simulink model "SIFT"  (R2013a)
settings: Solver=FixedStepDiscrete  SolverMode=SingleTasking  StartTime=0.0  StopTime=10.0  RelTol=1e-3
libraries: xbsIndex_r4 x365, xrbsImage_r4 x64
(part 1 of 10)
settings Model: Creator=Gururaja  LastModifiedBy=Gururaja
settings DataIOCC: SignalLogging=off
settings OptimizationCC: BlockReduction=off  ConditionallyExecuteInputs=off  InlineParams=on
settings DebuggingCC: AlgebraicLoopMsg=error
settings HardwareCC: ProdHWDeviceType=ASIC/FPGA->ASIC/FPGA  ProdEqTarget=off

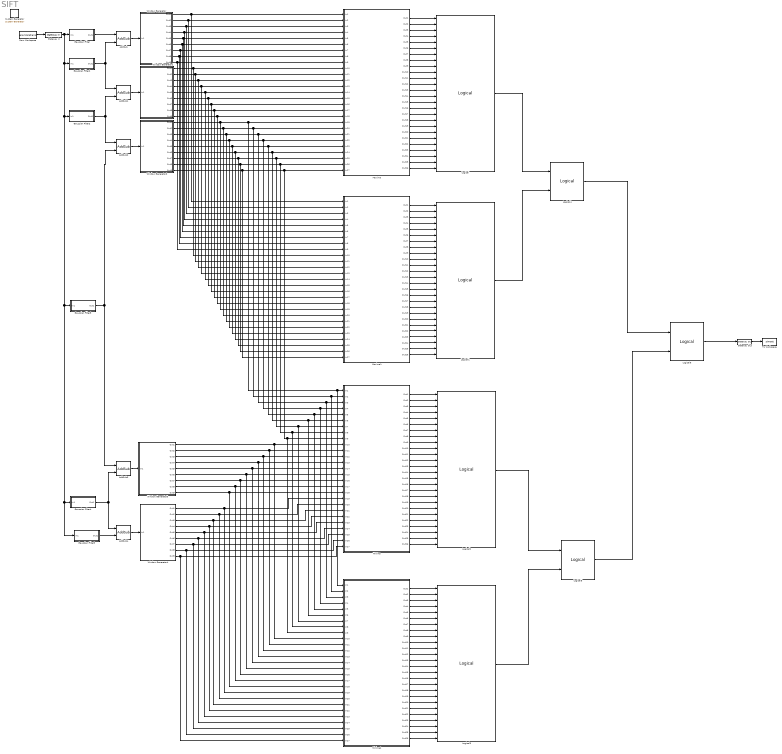
== system SIFT ==
  " System Generator" : xbsIndex_r4/ System Generator  Tag=genX  xilinxfamily=virtex5  part=xc5vsx50t  speed=-1  package=ff1136  synthesis_tool=XST  clock_wrapper=Clock Enables  directory=./netlist  proj_type=Project Navigator  Synth_file=XST Defaults  Impl_file=ISE Defaults  testbench=off  simulink_period=1  sysclk_period=10  dcm_input_clock_period=10  incr_netlist=off  trim_vbits=Everywhere in SubSystem  dbl_ovrd=According to Block Masks  core_generation=According to Block Masks  run_coregen=off  deprecated_control=off  eval_field=0  block_type=sysgen
  AddSub{,1..4} (5 alike) : xbsIndex_r4/AddSub  mode=Subtraction  use_carryin=off  use_carryout=off  en=off  latency=0  precision=User Defined  arith_type=Unsigned  n_bits=8  bin_pt=0  quantization="Round  (unbiased: +/- Inf)"  overflow=Saturate  dbl_ovrd=off  use_behavioral_HDL=off  hw_selection=Fabric  pipelined=off  block_type=addsub
  From Workspace : FromWorkspace  VariableName=grayScaleSignal  SampleTime=1  Interpolate=off  OutputAfterFinalValue=Setting to zero
  Gateway In : xbsIndex_r4/Gateway In  gui_display_data_type=Fixed-point  arith_type=Unsigned  n_bits=8  bin_pt=0  preci_type=Single  exp_width=8  frac_width=24  quantization="Round  (unbiased: +/- Inf)"  overflow=Saturate  period=1  dbl_ovrd=off  timing_constraint=None  locs_specified=off  LOCs={}  UseAsADC=off  ADCChannel='1'  inherit_from_input=off  hdl_port=on  block_type=gatewayin
  Gateway Out : xbsIndex_r4/Gateway Out  inherit_from_input=off  hdl_port=on  timing_constraint="Data Rate;  Set 'FAST' Attribute"  locs_specified=off  LOCs={}  UseAsDAC=off  DACChannel='1'  block_type=gatewayout
  Gaussian Filter : Subsystem
  Gaussian Filter1 : Subsystem
  Gaussian Filter2 : Subsystem
  Gaussian Filter3 : Subsystem
  Gaussian Filter4 : Subsystem
  Gaussian Filter5 : Subsystem
  Logical{,1..3} (4 alike) : xbsIndex_r4/Logical  logical_function=AND  inputs=26  en=off  latency=1  precision=User Defined  arith_type=Unsigned  n_bits=8  bin_pt=0  align_bp=on  dbl_ovrd=off  block_type=logical
  Logical4 : xbsIndex_r4/Logical  logical_function=OR  inputs=2  en=off  latency=1  precision=Full  arith_type=Unsigned  n_bits=16  bin_pt=0  align_bp=on  dbl_ovrd=off  block_type=logical
  Logical5 : xbsIndex_r4/Logical  logical_function=OR  inputs=2  en=off  latency=1  precision=Full  arith_type=Unsigned  n_bits=16  bin_pt=0  align_bp=on  dbl_ovrd=off  block_type=logical
  Logical6 : xbsIndex_r4/Logical  logical_function=OR  inputs=2  en=off  latency=1  precision=Full  arith_type=Unsigned  n_bits=16  bin_pt=0  align_bp=on  dbl_ovrd=off  block_type=logical
  Maxima : Subsystem
  Maxima1 : Subsystem
  Minima : Subsystem
  Minima1 : Subsystem
  To Workspace : ToWorkspace  VariableName=simout  SampleTime=1
  Window Generator : Subsystem
  Window Generator1 : Subsystem
  Window Generator2 : Subsystem
  Window Generator3 : Subsystem
  Window Generator4 : Subsystem
  wires:
  From Workspace/1 -> Gateway In/1
  Gateway In/1 -> Gaussian Filter1/1(In1), Gaussian Filter2/1(In1), Gaussian Filter3/1(In1), Gaussian Filter5/1(In1), Gaussian Filter4/1(In1), Gaussian Filter/1(In1)
  AddSub/1 -> Window Generator/1(In1)
  AddSub1/1 -> Window Generator1/1(In1)
  AddSub2/1 -> Window Generator2/1(In1)
  AddSub3/1 -> Window Generator3/1(In1)
  AddSub4/1 -> Window Generator4/1(In1)
  Window Generator/1(Out1) -> Maxima1/1(In1), Maxima/1(In1)
  Window Generator/3(Out3) -> Maxima1/3(In3), Maxima/3(In3)
  Window Generator/4(Out4) -> Maxima1/4(In4), Maxima/4(In4)
  Window Generator/5(Out5) -> Maxima1/5(In5), Maxima/5(In5)
  Window Generator/6(Out6) -> Maxima1/6(In6), Maxima/6(In6)
  Window Generator/7(Out7) -> Maxima1/7(In7), Maxima/7(In7)
  Window Generator/8(Out8) -> Maxima1/8(In8), Maxima/8(In8)
  Window Generator/9(Out9) -> Maxima1/9(In9), Maxima/9(In9)
  Window Generator1/1(Out1) -> Maxima1/10(In10), Maxima/10(In10)
  Window Generator1/2(Out2) -> Maxima1/11(In11), Maxima/11(In11)
  Window Generator1/3(Out3) -> Maxima1/12(In12), Maxima/12(In12)
  Window Generator1/4(Out4) -> Maxima1/13(In13), Maxima/13(In13)
  Window Generator1/5(Out5) -> Maxima1/14(In14), Maxima/14(In14)
  Window Generator1/6(Out6) -> Maxima1/15(In15), Maxima/15(In15)
  Window Generator1/7(Out7) -> Maxima1/16(In16), Maxima/16(In16)
  Window Generator1/8(Out8) -> Maxima1/17(In17), Maxima/17(In17)
  Window Generator1/9(Out9) -> Maxima1/18(In18), Maxima/18(In18)
  Window Generator2/1(Out1) -> Maxima1/19(In19), Minima1/1(In1), Minima/1(In1), Maxima/19(In19)
  Window Generator2/2(Out2) -> Maxima1/20(In20), Minima1/2(In2), Minima/2(In2), Maxima/20(In20)
  Window Generator2/3(Out3) -> Maxima1/21(In21), Minima1/3(In3), Minima/3(In3), Maxima/21(In21)
  Window Generator2/4(Out4) -> Maxima1/22(In22), Minima1/4(In4), Minima/4(In4), Maxima/22(In22)
  Window Generator2/5(Out5) -> Maxima1/23(In23), Minima1/5(In5), Minima/5(In5), Maxima/23(In23)
  Window Generator2/6(Out6) -> Maxima1/24(In24), Minima1/6(In6), Minima/6(In6), Maxima/24(In24)
  Window Generator2/7(Out7) -> Maxima1/25(In25), Minima1/7(In7), Minima/7(In7), Maxima/25(In25)
  Window Generator2/8(Out8) -> Maxima1/26(In26), Minima1/8(In8), Minima/8(In8), Maxima/26(In26)
  Window Generator2/9(Out9) -> Maxima1/27(In27), Minima1/9(In9), Minima/9(In9), Maxima/27(In27)
  Window Generator/2(Out2) -> Maxima1/2(In2), Maxima/2(In2)
  Window Generator3/1(Out1) -> Minima1/10(In10), Minima/10(In10)
  Window Generator3/2(Out2) -> Minima1/11(In11), Minima/11(In11)
  Window Generator3/3(Out3) -> Minima1/12(In12), Minima/12(In12)
  Window Generator3/4(Out4) -> Minima1/13(In13), Minima/13(In13)
  Window Generator3/5(Out5) -> Minima1/14(In14), Minima/14(In14)
  Window Generator3/6(Out6) -> Minima1/15(In15), Minima/15(In15)
  Window Generator3/7(Out7) -> Minima1/16(In16), Minima/16(In16)
  Window Generator3/8(Out8) -> Minima1/17(In17), Minima/17(In17)
  Window Generator3/9(Out9) -> Minima1/18(In18), Minima/18(In18)
  Window Generator4/1(Out1) -> Minima1/19(In19), Minima/19(In19)
  Window Generator4/2(Out2) -> Minima1/20(In20), Minima/20(In20)
  Window Generator4/3(Out3) -> Minima1/21(In21), Minima/21(In21)
  Window Generator4/4(Out4) -> Minima1/22(In22), Minima/22(In22)
  Window Generator4/5(Out5) -> Minima1/23(In23), Minima/23(In23)
  Window Generator4/6(Out6) -> Minima1/24(In24), Minima/24(In24)
  Window Generator4/7(Out7) -> Minima1/25(In25), Minima/25(In25)
  Window Generator4/8(Out8) -> Minima1/26(In26), Minima/26(In26)
  Window Generator4/9(Out9) -> Minima1/27(In27), Minima/27(In27)
  Maxima/1(Out1) -> Logical/1
  Maxima/2(Out2) -> Logical/2
  Maxima/3(Out3) -> Logical/3
  Maxima/4(Out4) -> Logical/4
  Maxima/5(Out5) -> Logical/5
  Maxima/6(Out6) -> Logical/6
  Maxima/7(Out7) -> Logical/7
  Maxima/8(Out8) -> Logical/8
  Maxima/9(Out9) -> Logical/9
  Maxima/10(Out10) -> Logical/10
  Maxima/11(Out11) -> Logical/11
  Maxima/12(Out12) -> Logical/12
  Maxima/13(Out13) -> Logical/13
  Maxima/14(Out14) -> Logical/14
  Maxima/15(Out15) -> Logical/15
  Maxima/16(Out16) -> Logical/16
  Maxima/17(Out17) -> Logical/17
  Maxima/18(Out18) -> Logical/18
  Maxima/19(Out19) -> Logical/19
  Maxima/20(Out20) -> Logical/20
  Maxima/21(Out21) -> Logical/21
  Maxima/22(Out22) -> Logical/22
  Maxima/23(Out23) -> Logical/23
  Maxima/24(Out24) -> Logical/24
  Maxima/25(Out25) -> Logical/25
  Maxima/26(Out26) -> Logical/26
  Maxima1/1(Out1) -> Logical1/1
  Maxima1/2(Out2) -> Logical1/2
  Maxima1/3(Out3) -> Logical1/3
  Maxima1/4(Out4) -> Logical1/4
  Maxima1/5(Out5) -> Logical1/5
  Maxima1/6(Out6) -> Logical1/6
  Maxima1/7(Out7) -> Logical1/7
  Maxima1/8(Out8) -> Logical1/8
  Maxima1/9(Out9) -> Logical1/9
  Maxima1/10(Out10) -> Logical1/10
  Maxima1/11(Out11) -> Logical1/11
  Maxima1/12(Out12) -> Logical1/12
  Maxima1/13(Out13) -> Logical1/13
  Maxima1/14(Out14) -> Logical1/14
  Maxima1/15(Out15) -> Logical1/15
  Maxima1/16(Out16) -> Logical1/16
  Maxima1/17(Out17) -> Logical1/17
  Maxima1/18(Out18) -> Logical1/18
  Maxima1/19(Out19) -> Logical1/19
  Maxima1/20(Out20) -> Logical1/20
  Maxima1/21(Out21) -> Logical1/21
  Maxima1/22(Out22) -> Logical1/22
  Maxima1/23(Out23) -> Logical1/23
  Maxima1/24(Out24) -> Logical1/24
  Maxima1/25(Out25) -> Logical1/25
  Maxima1/26(Out26) -> Logical1/26
  Minima/1(Out1) -> Logical2/1
  Minima/2(Out2) -> Logical2/2
  Minima/3(Out3) -> Logical2/3
  Minima/4(Out4) -> Logical2/4
  Minima/5(Out5) -> Logical2/5
  Minima/6(Out6) -> Logical2/6
  Minima/7(Out7) -> Logical2/7
  Minima/8(Out8) -> Logical2/8
  Minima/9(Out9) -> Logical2/9
  Minima/10(Out10) -> Logical2/10
  Minima/11(Out11) -> Logical2/11
  Minima/12(Out12) -> Logical2/12
  Minima/13(Out13) -> Logical2/13
  Minima/14(Out14) -> Logical2/14
  Minima/15(Out15) -> Logical2/15
  Minima/16(Out16) -> Logical2/16
  Minima/17(Out17) -> Logical2/17
  Minima/18(Out18) -> Logical2/18
  Minima/19(Out19) -> Logical2/19
  Minima/20(Out20) -> Logical2/20
  Minima/21(Out21) -> Logical2/21
  Minima/22(Out22) -> Logical2/22
  Minima/23(Out23) -> Logical2/23
  Minima/24(Out24) -> Logical2/24
  Minima/25(Out25) -> Logical2/25
  Minima/26(Out26) -> Logical2/26
  Minima1/1(Out1) -> Logical3/1
  Minima1/2(Out2) -> Logical3/2
  Minima1/3(Out3) -> Logical3/3
  Minima1/4(Out4) -> Logical3/4
  Minima1/5(Out5) -> Logical3/5
  Minima1/6(Out6) -> Logical3/6
  Minima1/7(Out7) -> Logical3/7
  Minima1/8(Out8) -> Logical3/8
  Minima1/9(Out9) -> Logical3/9
  Minima1/10(Out10) -> Logical3/10
  Minima1/11(Out11) -> Logical3/11
  Minima1/12(Out12) -> Logical3/12
  Minima1/13(Out13) -> Logical3/13
  Minima1/14(Out14) -> Logical3/14
  Minima1/15(Out15) -> Logical3/15
  Minima1/16(Out16) -> Logical3/16
  Minima1/17(Out17) -> Logical3/17
  Minima1/18(Out18) -> Logical3/18
  Minima1/19(Out19) -> Logical3/19
  Minima1/20(Out20) -> Logical3/20
  Minima1/21(Out21) -> Logical3/21
  Minima1/22(Out22) -> Logical3/22
  Minima1/23(Out23) -> Logical3/23
  Minima1/24(Out24) -> Logical3/24
  Minima1/25(Out25) -> Logical3/25
  Minima1/26(Out26) -> Logical3/26
  Logical/1 -> Logical4/1
  Logical1/1 -> Logical4/2
  Logical2/1 -> Logical5/1
  Logical3/1 -> Logical5/2
  Logical4/1 -> Logical6/1
  Logical5/1 -> Logical6/2
  Logical6/1 -> Gateway Out/1
  Gateway Out/1 -> To Workspace/1
  Gaussian Filter/1(Out1) -> AddSub/1
  Gaussian Filter1/1(Out1) -> AddSub/2, AddSub1/1
  Gaussian Filter2/1(Out1) -> AddSub2/1, AddSub1/2
  Gaussian Filter3/1(Out1) -> AddSub2/2, AddSub3/1
  Gaussian Filter4/1(Out1) -> AddSub4/1, AddSub3/2
  Gaussian Filter5/1(Out1) -> AddSub4/2

== system SIFT/Gaussian Filter ==
  In1 : Inport
  AddSub{,1..4} (5 alike) : xbsIndex_r4/AddSub  mode=Addition  use_carryin=off  use_carryout=off  en=off  latency=0  precision=Full  arith_type=Unsigned  n_bits=16  bin_pt=14  quantization=Truncate  overflow=Wrap  dbl_ovrd=off  use_behavioral_HDL=off  hw_selection=Fabric  pipelined=off  block_type=addsub
  Delay : xbsIndex_r4/Delay  rst=off  infoeditControl=Selection of Reset will increase slice count due to use of real FFs and instead of SRLs  en=off  latency=1  dbl_ovrd=off  reg_retiming=off  block_type=delay
  Subsystem : Subsystem
  Virtex Line Buffer : xrbsImage_r4/Virtex Line Buffer  buf_depth=720  cst=1
  Virtex2 Line Buffer : xrbsImage_r4/Virtex2 Line Buffer  buf_depth=720  cst=1
      link override Single Port RAM: block_version=8.2
  Virtex2 Line Buffer1 : xrbsImage_r4/Virtex2 Line Buffer  buf_depth=720  cst=1
      link override Single Port RAM: block_version=8.2
  Virtex2 Line Buffer2 : xrbsImage_r4/Virtex2 Line Buffer  buf_depth=720  cst=1
      link override Single Port RAM: block_version=8.2
  Out1 : Outport
  wires:
  In1/1 -> Subsystem/1(In1), Virtex Line Buffer/1
  Virtex Line Buffer/1 -> Virtex2 Line Buffer/1, Subsystem/2(In2)
  Virtex2 Line Buffer/1 -> Virtex2 Line Buffer1/1, Subsystem/3(In3)
  Virtex2 Line Buffer1/1 -> Subsystem/4(In4), Virtex2 Line Buffer2/1
  Virtex2 Line Buffer2/1 -> Subsystem/5(In5)
  Subsystem/1(Out1) -> AddSub/1
  Subsystem/2(Out2) -> AddSub/2
  Subsystem/3(Out3) -> AddSub1/1
  Subsystem/4(Out4) -> AddSub1/2
  Subsystem/5(Out5) -> AddSub2/1
  Subsystem/6(Out6) -> AddSub2/2
  AddSub/1 -> AddSub3/1
  AddSub1/1 -> AddSub3/2
  AddSub2/1 -> Delay/1
  Delay/1 -> AddSub4/2
  AddSub3/1 -> AddSub4/1
  AddSub4/1 -> Out1/1

== system SIFT/Gaussian Filter1 ==
  In1 : Inport
  AddSub{,1..4} (5 alike) : xbsIndex_r4/AddSub  mode=Addition  use_carryin=off  use_carryout=off  en=off  latency=0  precision=Full  arith_type=Unsigned  n_bits=16  bin_pt=14  quantization=Truncate  overflow=Wrap  dbl_ovrd=off  use_behavioral_HDL=off  hw_selection=Fabric  pipelined=off  block_type=addsub
  Delay : xbsIndex_r4/Delay  rst=off  infoeditControl=Selection of Reset will increase slice count due to use of real FFs and instead of SRLs  en=off  latency=1  dbl_ovrd=off  reg_retiming=off  block_type=delay
  Subsystem : Subsystem
  Virtex Line Buffer : xrbsImage_r4/Virtex Line Buffer  buf_depth=720  cst=1
  Virtex2 Line Buffer : xrbsImage_r4/Virtex2 Line Buffer  buf_depth=720  cst=1
      link override Single Port RAM: block_version=8.2
  Virtex2 Line Buffer1 : xrbsImage_r4/Virtex2 Line Buffer  buf_depth=720  cst=1
      link override Single Port RAM: block_version=8.2
  Virtex2 Line Buffer2 : xrbsImage_r4/Virtex2 Line Buffer  buf_depth=720  cst=1
      link override Single Port RAM: block_version=8.2
  Out1 : Outport
  wires:
  In1/1 -> Subsystem/1(In1), Virtex Line Buffer/1
  Virtex Line Buffer/1 -> Virtex2 Line Buffer/1, Subsystem/2(In2)
  Virtex2 Line Buffer/1 -> Virtex2 Line Buffer1/1, Subsystem/3(In3)
  Virtex2 Line Buffer1/1 -> Subsystem/4(In4), Virtex2 Line Buffer2/1
  Virtex2 Line Buffer2/1 -> Subsystem/5(In5)
  Subsystem/1(Out1) -> AddSub/1
  Subsystem/2(Out2) -> AddSub/2
  Subsystem/3(Out3) -> AddSub1/1
  Subsystem/4(Out4) -> AddSub1/2
  Subsystem/5(Out5) -> AddSub2/1
  Subsystem/6(Out6) -> AddSub2/2
  AddSub/1 -> AddSub3/1
  AddSub1/1 -> AddSub3/2
  AddSub2/1 -> Delay/1
  Delay/1 -> AddSub4/2
  AddSub3/1 -> AddSub4/1
  AddSub4/1 -> Out1/1

== system SIFT/Gaussian Filter2 ==
  In1 : Inport
  AddSub{,1..4} (5 alike) : xbsIndex_r4/AddSub  mode=Addition  use_carryin=off  use_carryout=off  en=off  latency=0  precision=Full  arith_type=Unsigned  n_bits=16  bin_pt=14  quantization=Truncate  overflow=Wrap  dbl_ovrd=off  use_behavioral_HDL=off  hw_selection=Fabric  pipelined=off  block_type=addsub
  Delay : xbsIndex_r4/Delay  rst=off  infoeditControl=Selection of Reset will increase slice count due to use of real FFs and instead of SRLs  en=off  latency=1  dbl_ovrd=off  reg_retiming=off  block_type=delay
  Subsystem : Subsystem
  Virtex Line Buffer : xrbsImage_r4/Virtex Line Buffer  buf_depth=720  cst=1
  Virtex2 Line Buffer : xrbsImage_r4/Virtex2 Line Buffer  buf_depth=720  cst=1
      link override Single Port RAM: block_version=8.2
  Virtex2 Line Buffer1 : xrbsImage_r4/Virtex2 Line Buffer  buf_depth=720  cst=1
      link override Single Port RAM: block_version=8.2
  Virtex2 Line Buffer2 : xrbsImage_r4/Virtex2 Line Buffer  buf_depth=720  cst=1
      link override Single Port RAM: block_version=8.2
  Out1 : Outport
  wires:
  In1/1 -> Subsystem/1(In1), Virtex Line Buffer/1
  Virtex Line Buffer/1 -> Virtex2 Line Buffer/1, Subsystem/2(In2)
  Virtex2 Line Buffer/1 -> Virtex2 Line Buffer1/1, Subsystem/3(In3)
  Virtex2 Line Buffer1/1 -> Subsystem/4(In4), Virtex2 Line Buffer2/1
  Virtex2 Line Buffer2/1 -> Subsystem/5(In5)
  Subsystem/1(Out1) -> AddSub/1
  Subsystem/2(Out2) -> AddSub/2
  Subsystem/3(Out3) -> AddSub1/1
  Subsystem/4(Out4) -> AddSub1/2
  Subsystem/5(Out5) -> AddSub2/1
  Subsystem/6(Out6) -> AddSub2/2
  AddSub/1 -> AddSub3/1
  AddSub1/1 -> AddSub3/2
  AddSub2/1 -> Delay/1
  Delay/1 -> AddSub4/2
  AddSub3/1 -> AddSub4/1
  AddSub4/1 -> Out1/1
